simulink subsystem "Vehicle_Sim"  (R2020b)
settings: Solver=VariableStepAuto  StartTime=0.0  StopTime=10.0  RelTol=1e-3
settings Model: Creator=rthom  LastModifiedBy=david

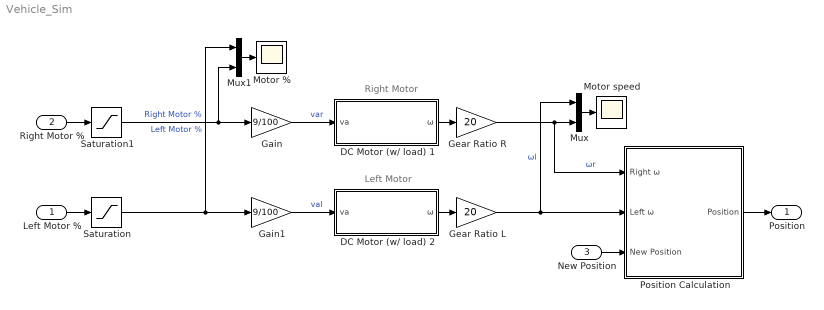
== system Vehicle_Sim ==
  note: Right Motor
  note: Left Motor
  Left Motor % : Inport
  Right Motor % : Inport  Port=2
  New Position : Inport  Port=3
  DC Motor (w/ load) 1 : Subsystem
  DC Motor (w/ load) 2 : Subsystem
  Gain : Gain  Gain=9/100
  Gain1 : Gain  Gain=9/100
  Gear Ratio L : Gain  Gain=20
  Gear Ratio R : Gain  Gain=20
  Motor % : Scope
  Motor speed : Scope
  Mux : Mux  Inputs=2
  Mux1 : Mux  Inputs=2
  Position Calculation : Subsystem
  Saturation : Saturate  UpperLimit=100  LowerLimit=-100
  Saturation1 : Saturate  UpperLimit=100  LowerLimit=-100
  Position : Outport
  wires:
  Gear Ratio R/1 -> Mux/2, Position Calculation/1(Right ω)  "ωr"
  Gear Ratio L/1 -> Mux/1, Position Calculation/2(Left ω)  "ωl"
  Mux/1 -> Motor speed/1
  Mux1/1 -> Motor %/1
  Saturation1/1 -> Gain/1, Mux1/2  "Right Motor %"
  Saturation/1 -> Mux1/1, Gain1/1  "Left Motor %"
  Left Motor %/1 -> Saturation/1
  Right Motor %/1 -> Saturation1/1
  DC Motor (w/ load) 1/1(ω) -> Gear Ratio R/1
  Gain/1 -> DC Motor (w/ load) 1/1(va)  "var"
  DC Motor (w/ load) 2/1(ω) -> Gear Ratio L/1
  Gain1/1 -> DC Motor (w/ load) 2/1(va)  "val"
  New Position/1 -> Position Calculation/3(New Position)
  Position Calculation/1(Position) -> Position/1

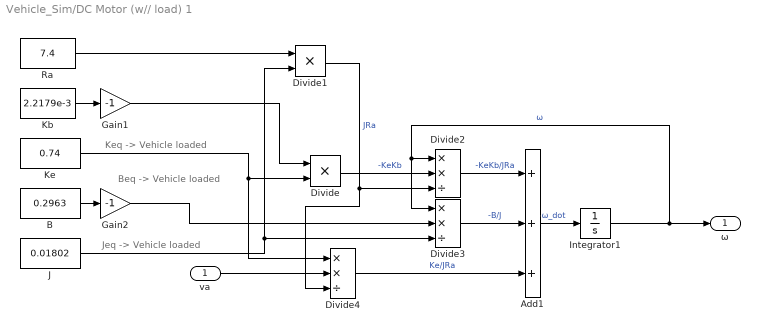
== system Vehicle_Sim/DC Motor (w// load) 1 ==
  note: Keq -> Vehicle loaded
  note: Beq -> Vehicle loaded
  note: Jeq -> Vehicle loaded
  va : Inport
  Add1 : Sum  Inputs=+++
  B : Constant  Value=0.2963
  Divide : Product  Inputs=**
  Divide1 : Product  Inputs=**
  Divide2 : Product  Inputs=**/
  Divide3 : Product  Inputs=**/
  Divide4 : Product  Inputs=**/
  Gain1 : Gain  Gain=-1
  Gain2 : Gain  Gain=-1
  Integrator1 : Integrator
  J : Constant  Value=0.01802
  Kb : Constant  Value=2.2179e-3
  Ke : Constant  Value=0.74
  Ra : Constant  Value=7.4
  ω : Outport
  wires:
  va/1 -> Divide4/2
  Integrator1/1 -> Divide3/1, Divide2/1, ω/1  "ω"
  Divide4/1 -> Add1/3  "Ke/JRa"
  Divide/1 -> Divide2/2  "-KeKb"
  Divide1/1 -> Divide2/3, Divide4/3  "JRa"
  Gain1/1 -> Divide/1
  Divide3/1 -> Add1/2  "-B/J"
  Gain2/1 -> Divide3/2
  J/1 -> Divide1/2, Divide3/3
  Ra/1 -> Divide1/1
  Ke/1 -> Divide4/1, Divide/2
  Kb/1 -> Gain1/1
  Add1/1 -> Integrator1/1  "ω_dot"
  Divide2/1 -> Add1/1  "-KeKb/JRa"
  B/1 -> Gain2/1

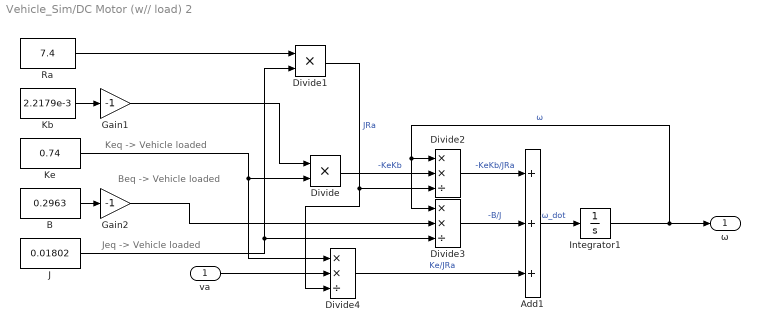
== system Vehicle_Sim/DC Motor (w// load) 2 ==
  note: Keq -> Vehicle loaded
  note: Beq -> Vehicle loaded
  note: Jeq -> Vehicle loaded
  va : Inport
  Add1 : Sum  Inputs=+++
  B : Constant  Value=0.2963
  Divide : Product  Inputs=**
  Divide1 : Product  Inputs=**
  Divide2 : Product  Inputs=**/
  Divide3 : Product  Inputs=**/
  Divide4 : Product  Inputs=**/
  Gain1 : Gain  Gain=-1
  Gain2 : Gain  Gain=-1
  Integrator1 : Integrator
  J : Constant  Value=0.01802
  Kb : Constant  Value=2.2179e-3
  Ke : Constant  Value=0.74
  Ra : Constant  Value=7.4
  ω : Outport
  wires:
  va/1 -> Divide4/2
  Integrator1/1 -> Divide3/1, Divide2/1, ω/1  "ω"
  Divide4/1 -> Add1/3  "Ke/JRa"
  Divide/1 -> Divide2/2  "-KeKb"
  Divide1/1 -> Divide2/3, Divide4/3  "JRa"
  Gain1/1 -> Divide/1
  Divide3/1 -> Add1/2  "-B/J"
  Gain2/1 -> Divide3/2
  J/1 -> Divide1/2, Divide3/3
  Ra/1 -> Divide1/1
  Ke/1 -> Divide4/1, Divide/2
  Kb/1 -> Gain1/1
  Add1/1 -> Integrator1/1  "ω_dot"
  Divide2/1 -> Add1/1  "-KeKb/JRa"
  B/1 -> Gain2/1

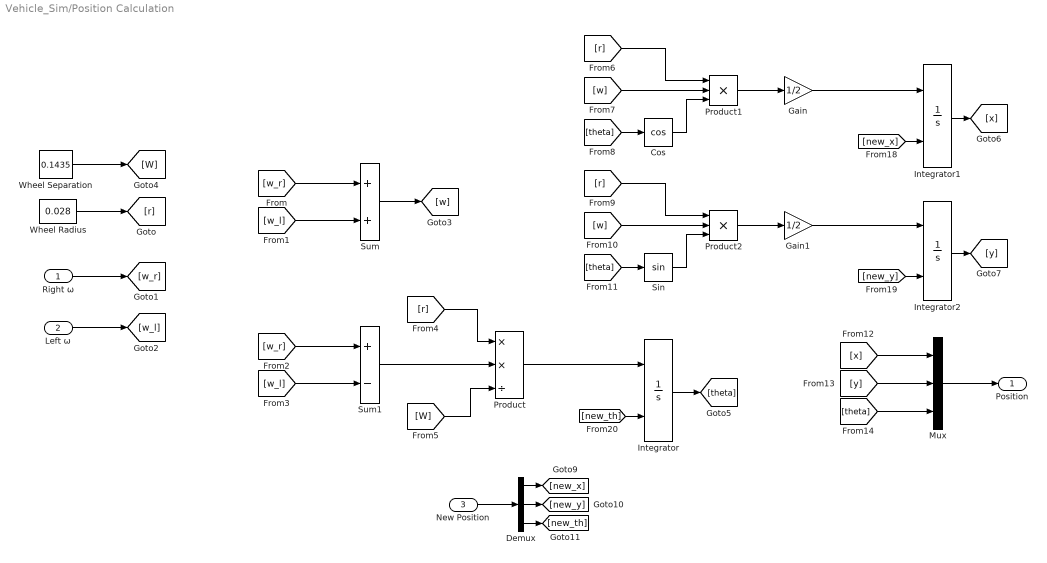
== system Vehicle_Sim/Position Calculation ==
  Right ω : Inport
  Left ω : Inport  Port=2
  New Position : Inport  Port=3
  Cos : Trigonometry  Operator=cos
  Demux : Demux  Outputs=3
  Gain : Gain  Gain=1/2
  Gain1 : Gain  Gain=1/2
  Integrator : Integrator  InitialConditionSource=external
  Integrator1 : Integrator  InitialConditionSource=external
  Integrator2 : Integrator  InitialConditionSource=external
  Mux : Mux  Inputs=3
  Product : Product  Inputs=**/
  Product1 : Product  Inputs=3
  Product2 : Product  Inputs=3
  Sin : Trigonometry
  Sum : Sum
  Sum1 : Sum  Inputs=+-
  Wheel Radius : Constant  Value=0.028
  Wheel Separation : Constant  Value=0.1435
  Position : Outport
  wires:
  Mux/1 -> Position/1
  [y] -> Mux/2
  [x] -> Mux/1
  Integrator1/1 -> [x]
  Gain/1 -> Integrator1/1
  [theta] -> Cos/1
  Integrator2/1 -> [y]
  [new_y] -> Integrator2/2
  Demux/3 -> [new_th]
  Gain1/1 -> Integrator2/1
  [theta] -> Sin/1
  [r] -> Product1/1
  Right ω/1 -> [w_r]
  [w_r] -> Sum1/1
  Product/1 -> Integrator/1
  Integrator/1 -> [theta]
  [r] -> Product/1
  Product1/1 -> Gain/1
  [w] -> Product2/2
  [r] -> Product2/1
  [w] -> Product1/2
  [W] -> Product/3
  [w_l] -> Sum1/2
  Sum1/1 -> Product/2
  Cos/1 -> Product1/3
  [theta] -> Mux/3
  Left ω/1 -> [w_l]
  Wheel Separation/1 -> [W]
  [w_r] -> Sum/1
  Sin/1 -> Product2/3
  New Position/1 -> Demux/1
  Sum/1 -> [w]
  [w_l] -> Sum/2
  Demux/2 -> [new_y]
  Demux/1 -> [new_x]
  Wheel Radius/1 -> [r]
  [new_x] -> Integrator1/2
  Product2/1 -> Gain1/1
  [new_th] -> Integrator/2
